simulink model "sliding_goertzel_model"  (R2019b)
settings: Solver=VariableStepAuto  StartTime=0.0  StopTime=10.0  RelTol=1e-3
settings Model: Creator=jozef  LastModifiedBy=jozef

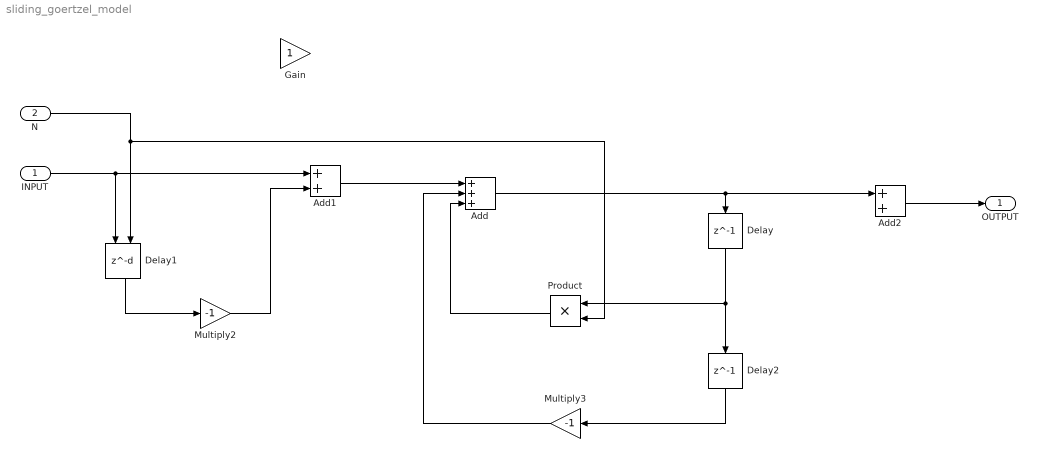
== system sliding_goertzel_model ==
  INPUT : Inport
  N : Inport  Port=2
  Add : Sum  Inputs=+++
  Add1 : Sum
  Add2 : Sum
  Delay : Delay  DelayLength=1  InitialCondition=0
  Delay1 : Delay  DelayLengthSource=Input port  DelayLength=1  InitialCondition=0
      settings: InputPortMap=u0,p1
  Delay2 : Delay  DelayLength=1  InitialCondition=0
  Gain : Gain
  Multiply2 : Gain  Gain=-1
  Multiply3 : Gain  Gain=-1
  Product : Product
  "OUTPUT " : Outport
  wires:
  INPUT/1 -> Add1/1, Delay1/1
  Delay1/1 -> Multiply2/1
  Multiply2/1 -> Add1/2
  Add1/1 -> Add/1
  Delay/1 -> Product/1, Delay2/1
  Delay2/1 -> Multiply3/1
  Add/1 -> Add2/1, Delay/1
  Add2/1 -> "OUTPUT "/1
  Multiply3/1 -> Add/2
  Product/1 -> Add/3
  N/1 -> Product/2, Delay1/2
